simulink model "TractiveSystemTemperatures"  (R2024b)
settings: configuration reference "STM32H7_Config" (kept outside this file)
settings Model: DataDictionary=Master_Dictionary.sldd  EnableAccessToBaseWorkspace=off  Creator=torni  LastModifiedBy=William
settings ConfigSetRef: SourceName=STM32H7_Config

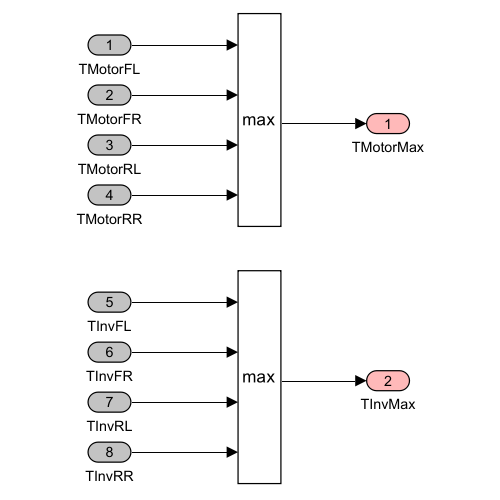
[thumbnail: Simulink's stored preview of the top-level diagram]
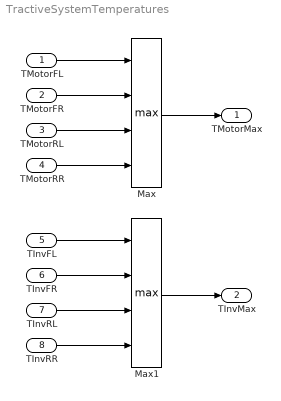
== system TractiveSystemTemperatures ==
  TMotorFL : Inport  OutDataTypeStr=double
  "TMotorFR " : Inport  Port=2  OutDataTypeStr=double
  TMotorRL : Inport  Port=3  OutDataTypeStr=double
  TMotorRR : Inport  Port=4  OutDataTypeStr=double
  TInvFL : Inport  Port=5  OutDataTypeStr=double
  TInvFR : Inport  Port=6  OutDataTypeStr=double
  TInvRL : Inport  Port=7  OutDataTypeStr=double
  TInvRR : Inport  Port=8  OutDataTypeStr=double
  Max : MinMax  Function=max  Inputs=4
  Max1 : MinMax  Function=max  Inputs=4
  TMotorMax : Outport  OutDataTypeStr=double  VectorParamsAs1DForOutWhenUnconnected=off
  TInvMax : Outport  Port=2  OutDataTypeStr=double  VectorParamsAs1DForOutWhenUnconnected=off
  wires:
  TMotorFL/1 -> Max/1
  TMotorRR/1 -> Max/4
  TMotorRL/1 -> Max/3
  "TMotorFR "/1 -> Max/2
  Max/1 -> TMotorMax/1
  Max1/1 -> TInvMax/1
  TInvFR/1 -> Max1/2
  TInvRL/1 -> Max1/3
  TInvRR/1 -> Max1/4
  TInvFL/1 -> Max1/1
